simulink model "task_1_regs_x"  (R2021b)
settings: Solver=FixedStepAuto  StartTime=0.0  StopTime=2  FixedStep=0.00005  RelTol=1e-3
settings Model: Creator=den  LastModifiedBy=den

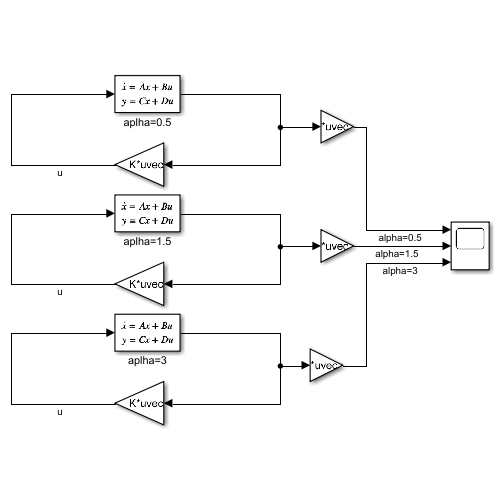
[thumbnail: Simulink's stored preview of the top-level diagram]
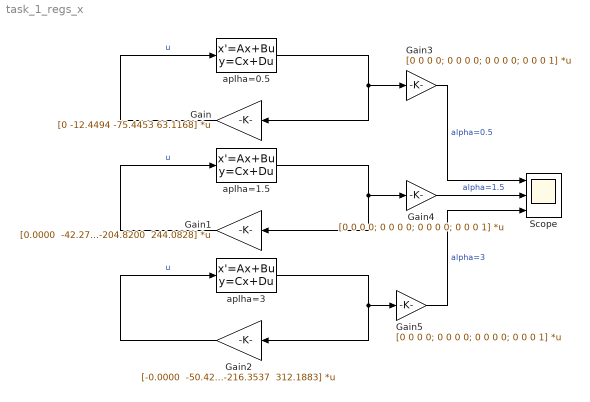
== system task_1_regs_x ==
  Gain : Gain  Gain=[0 -12.4494 -75.4453 63.1168]  Multiplication=Matrix(K*u) (u vector)
  Gain1 : Gain  Gain="[0.0000  -42.2752 -204.8200  244.0828]"  Multiplication=Matrix(K*u) (u vector)
  Gain2 : Gain  Gain="[-0.0000  -50.4259 -216.3537  312.1883]"  Multiplication=Matrix(K*u) (u vector)
  Gain3 : Gain  Gain=[0 0 0 0; 0 0 0 0; 0 0 0 0; 0 0 0 1]  Multiplication=Matrix(K*u) (u vector)
  Gain4 : Gain  Gain=[0 0 0 0; 0 0 0 0; 0 0 0 0; 0 0 0 1]  Multiplication=Matrix(K*u) (u vector)
  Gain5 : Gain  Gain=[0 0 0 0; 0 0 0 0; 0 0 0 0; 0 0 0 1]  Multiplication=Matrix(K*u) (u vector)
  Scope : Scope  NumInputPorts=3
  aplha=0.5 : StateSpace  A=[-3 0 0 0; 0 3 0 0; 0 0 3 3; 0 0 -3 3]  B=[0; 7; 0; 1]  C=[1 0 0 0; 0 1 0 0; 0 0 1 0; 0 0 0 1]  D=[0; 0; 0; 0]  InitialCondition=[-3; 17; 2; -8]
  aplha=1.5 : StateSpace  A=[-3 0 0 0; 0 3 0 0; 0 0 3 3; 0 0 -3 3]  B=[0; 7; 0; 1]  C=[1 0 0 0; 0 1 0 0; 0 0 1 0; 0 0 0 1]  D=[0; 0; 0; 0]  InitialCondition=[-3; 17; 2; -8]
  aplha=3 : StateSpace  A=[-3 0 0 0; 0 3 0 0; 0 0 3 3; 0 0 -3 3]  B=[0; 7; 0; 1]  C=[1 0 0 0; 0 1 0 0; 0 0 1 0; 0 0 0 1]  D=[0; 0; 0; 0]  InitialCondition=[-3; 17; 2; -8]
  wires:
  aplha=0.5/1 -> Gain/1, Gain3/1
  Gain/1 -> aplha=0.5/1  "u"
  Gain1/1 -> aplha=1.5/1  "u"
  aplha=1.5/1 -> Gain1/1, Gain4/1
  Gain2/1 -> aplha=3/1  "u"
  aplha=3/1 -> Gain5/1, Gain2/1
  Gain3/1 -> Scope/1  "alpha=0.5"
  Gain4/1 -> Scope/2  "alpha=1.5"
  Gain5/1 -> Scope/3  "alpha=3"
